simulink model "Genpath_simulink"  (R2018b)
settings: Solver=VariableStepAuto  StartTime=0.0  StopTime=0.8  RelTol=1e-3
values from neighbouring files (symbols this model uses):
  k = 350    [Genpath_program.m]    (also in Genpath_program_final.m)
  Kt = 0.048    [Genpath_program.m]    (also in Genpath_program_final.m)
  L = 10^-3    (= 0.001)    [Genpath_program.m]    (also in Genpath_program_final.m)
  M = m+Jp/(r2^2)+Jg/(r1^2)    (= 0.171805555556)    [Genpath_program.m]    (also in Genpath_program_final.m)
  r1 = 0.75*10^-2    (= 0.0075)    [Genpath_program.m]    (also in Genpath_program_final.m)
  RG = 50    [Genpath_program.m]    (also in Genpath_program_final.m)
  RL = Rd(i)    [Genpath_program.m]    (also in Genpath_program_final.m = Rd(i+1))
undefined symbols (not defined in the file or in its folder): sigbuilder_block
settings Model: Creator=Jzeta  LastModifiedBy=Jzeta

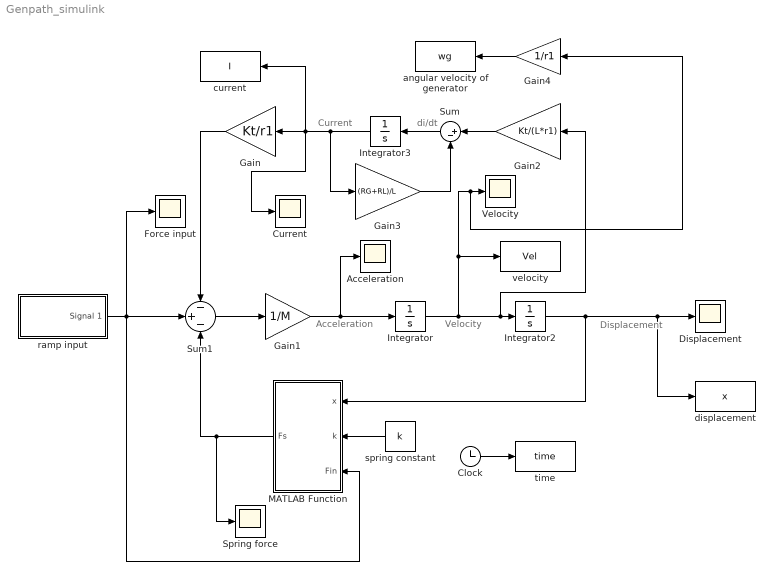
== system Genpath_simulink ==
  note: Current
  note: Acceleration
  note: Displacement
  note: Velocity
  note: di/dt
  Acceleration : Scope
  Clock : Clock
  Current : Scope
  Displacement : Scope
  Force input : Scope
  Gain : Gain  Gain=Kt/r1
  Gain1 : Gain  Gain=1/M
  Gain2 : Gain  Gain=Kt/(L*r1)
  Gain3 : Gain  Gain=(RG+RL)/L
  Gain4 : Gain  Gain=1/r1
  Integrator : Integrator
  Integrator2 : Integrator
  Integrator3 : Integrator
  MATLAB Function : MATLAB Function  TreatAsAtomicUnit=on
  Spring force : Scope
  Sum : Sum  Inputs=|+-
  Sum1 : Sum  Inputs=-+-
  Velocity : Scope
  angular velocity of generator : ToWorkspace  VariableName=wg  SampleTime=-1
  current : ToWorkspace  VariableName=I  SampleTime=-1
  displacement : ToWorkspace  VariableName=x  SampleTime=-1
  ramp input : Subsystem  Tag=STV Subsys  LoadFcn=sigbuilder_block('load');  StartFcn=sigbuilder_block('start');  StopFcn=sigbuilder_block('stop');  ClipboardFcn=sigbuilder_block('clipboard');  mask(Sigbuilder block){tuvar=[0:10]}
      mask help: Simulink:masks:SigbuilderBlock_MD
      mask init:
      | if ~strcmp(get_param(bdroot(gcbh),'SimulationStatus'),'stopped') tuvar = sigbuilder_block('maskInit'); end
      settings: CopyFcn=sigbuilder_block('copy');  DeleteFcn=sigbuilder_block('delete');  ModelCloseFcn=sigbuilder_block('modelClose');  PreSaveFcn=sigbuilder_block('preSave');  PauseFcn=sigbuilder_block('pause');  ContinueFcn=sigbuilder_block('continue');  NameChangeFcn=sigbuilder_block('namechange');  OpenFcn=sigbuilder_block('open',[437.6 153 550.4 359.25 ]);  CloseFcn=sigbuilder_block('close');
      mask Display: plot(0, 0, 100, 100,[2, 2, 32, 32, 2], [68, 8, 8, 68, 68],[32, 2], [38, 38], [32, 19, 2],[53, 60, 44], [32, 17, 17, 2],[16, 16, 31, 31]);txt = getActiveGroup(gcbh);text(2, 100, txt,'verticalAlignment', 'top');
  spring constant : Constant  Value=k
  time : ToWorkspace  VariableName=time  SampleTime=-1
  velocity : ToWorkspace  VariableName=Vel  SampleTime=-1
  wires:
  ramp input/1(Signal 1) -> Force input/1, MATLAB Function/3(Fin), Sum1/2
  MATLAB Function/1(Fs) -> Sum1/3, Spring force/1
  Gain/1 -> Sum1/1
  Sum1/1 -> Gain1/1
  Gain1/1 -> Acceleration/1, Integrator/1
  Integrator/1 -> velocity/1, Gain4/1, Velocity/1, Gain2/1, Integrator2/1
  Integrator2/1 -> MATLAB Function/1(x), Displacement/1, displacement/1
  Gain2/1 -> Sum/1
  Sum/1 -> Integrator3/1
  Integrator3/1 -> Gain3/1, Gain/1, current/1, Current/1
  Clock/1 -> time/1
  Gain3/1 -> Sum/2
  Gain4/1 -> angular velocity of generator/1
  spring constant/1 -> MATLAB Function/2(k)

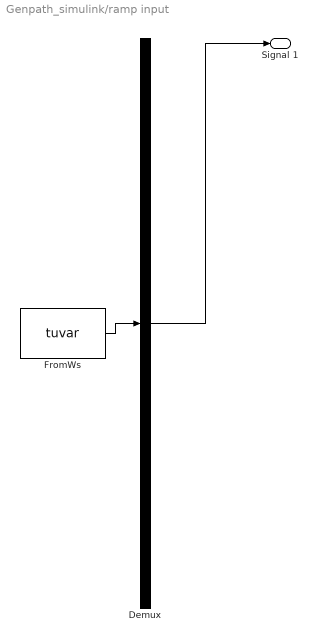
== system Genpath_simulink/ramp input ==
  Demux : Demux  Tag=STV Demux  Outputs=1
  FromWs : FromWorkspace  Tag=STV FromWs  VariableName=tuvar  SampleTime=0
      SigBuilderData=|
      | common.afterFinalStr = 'Extrapolate'
      | common.sampleTime = 0
      | dataSet.timeRange = [0 10]
      | dataSet.name = 'Group 1'
      | sbobj.Groups.Name = 'Group 1'
      | sbobj.Groups.Signals.Name = 'Signal 1'
      | sbobj.Groups.Signals.XData = [0 0.8 0.8 4 10]
      | sbobj.Groups.Signals.YData = [0 600 0 0 0]
  Signal 1 : Outport  Tag=STV Outport
  wires:
  Demux/1 -> Signal 1/1
  FromWs/1 -> Demux/1

== matlab function Genpath_simulink/MATLAB Function ==
  data: x input; k input; Fs output; Fin input
function Fs = fcn(x,k,Fin)
if x<0.02
    Fs = k*x;
else
    Fs = Fin;
end
